simulink model "ControlSystemDesign"  (R2020a)
settings: Solver=VariableStepAuto  StartTime=0.0  StopTime=100.0  RelTol=1e-3
values from neighbouring files (symbols this model uses):
  J = m/12*(l^2*cos(beta)^2+d^2*sin(beta)^2+w^2)    [SolarPanelMotorParams.m]
  Kd = 5    [SolarPanelMotorParams.m]
  Kf = 0.07    [SolarPanelMotorParams.m]
  Kg = 2000    [SolarPanelMotorParams.m]
  Kt = 0.07    [SolarPanelMotorParams.m]
  L = 1e-5    (= 1e-05)    [SolarPanelMotorParams.m]
  R = 10    [SolarPanelMotorParams.m]
libraries: simulink x1
settings Model: Creator=aztaa  LastModifiedBy=aztaa

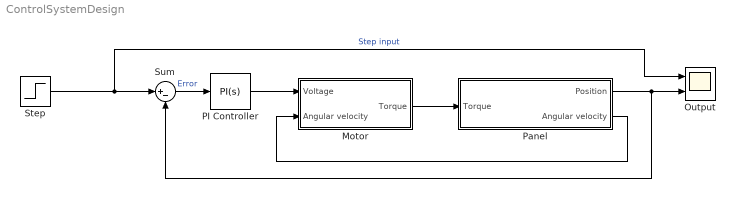
== system ControlSystemDesign ==
  Motor : Subsystem
  Output : Scope  NumInputPorts=2
  PI Controller : simulink/Continuous/PID Controller  Controller=PI  Form=Parallel  TimeDomain=Continuous-time  UseExternalTs=off  SampleTime=-1  IntegratorMethod=Forward Euler  FilterMethod=Forward Euler  ControllerParametersSource=internal  P=300  I=200  D=0  UseFilter=on  N=100  TunerSelectOption=Transfer Function Based (PID Tuner App)  InitialConditionSource=internal  InitialConditionForIntegrator=0  InitialConditionForFilter=0  DifferentiatorICPrevScaledInput=0  ExternalReset=none  TrackingMode=off  Kt=1  LimitOutput=off  UpperSaturationLimit=inf  LowerSaturationLimit=-inf  LinearizeAsGain=on  AntiWindupMode=none  Kb=1  POutMin=[]  POutMax=[]  IOutMin=[]  IOutMax=[]  DOutMin=[]  DOutMax=[]  NOutMin=[]  NOutMax=[]  SumOutMin=[]  SumOutMax=[]  SaturationOutMin=[]  SaturationOutMax=[]  PParamMin=[]  PParamMax=[]  IParamMin=[]  IParamMax=[]  DParamMin=[]  DParamMax=[]  NParamMin=[]  NParamMax=[]  KbParamMin=[]  KbParamMax=[]  KtParamMin=[]  KtParamMax=[]  KbOutMin=[]  KbOutMax=[]  KtOutMin=[]  KtOutMax=[]  IntegratorOutMin=[]  IntegratorOutMax=[]  FilterOutMin=[]  FilterOutMax=[]  SumI1OutMin=[]  SumI1OutMax=[]  SumI2OutMin=[]  SumI2OutMax=[]  SumI3OutMin=[]  SumI3OutMax=[]  SumI4OutMin=[]  SumI4OutMax=[]  SumDOutMin=[]  SumDOutMax=[]  DifferentiatorOutMin=[]  DifferentiatorOutMax=[]  FilterDiffOutCoefMin=[]  FilterDiffOutCoefMax=[]  ReciprocalOutMin=[]  ReciprocalOutMax=[]  SumDenOutMin=[]  SumDenOutMax=[]  SumNumOutMin=[]  SumNumOutMax=[]  DivideOutMin=[]  DivideOutMax=[]  UdiffTsProdOutMin=[]  UdiffTsProdOutMax=[]  NTsProdOutMin=[]  NTsProdOutMax=[]  UintegralTsProdOutMin=[]  UintegralTsProdOutMax=[]  UngainTsProdOutMin=[]  UngainTsProdOutMax=[]  IntegratorContinuousStateAttributes=''  IntegratorStateMustResolveToSignalObject=off  IntegratorRTWStateStorageClass=Auto  FilterContinuousStateAttributes=''  FilterStateMustResolveToSignalObject=off  FilterRTWStateStorageClass=Auto  ParallelPVariant=InternalParameters  IdealPVariant=Disabled  IVariant=InternalParameters  DVariant=Disabled  IntegratorVariant=Continuous  SatVariant=Disabled  AWVariant=Passthrough  PCopyVariant=Disabled  TRVariant=Disabled  FdbkBlocksVariant=Forward  IdealPFdbkVariant=Disabled  SatFdbkVariant=Disabled  DerivativeFilterVariant=Disabled  NVariant=Disabled  NCopyVariant=Disabled_SignalSpec  FilterICVariant=Disabled  IntegratorICVariant=InternalICs  ExternalResetVariant=Disabled  TRSumVariant=Passthrough  SumFdbkVariant=Disabled  SumVariant=Sum_PI  TsampFilterVariant=InternalTs  TsampNgainVariant=Passthrough  TsampIntegralVariant=Passthrough
  Panel : Subsystem
  Step : Step  SampleTime=0
  Sum : Sum  Inputs=|+-
  wires:
  Panel/1(Position) -> Output/2, Sum/2
  Motor/1(Torque) -> Panel/1(Torque)
  Panel/2(Angular velocity) -> Motor/2(Angular velocity)
  PI Controller/1 -> Motor/1(Voltage)
  Sum/1 -> PI Controller/1  "Error"
  Step/1 -> Output/1, Sum/1  "Step input"

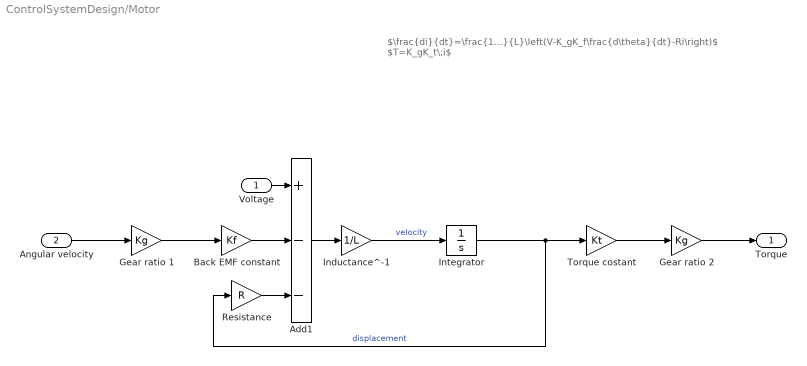
== system ControlSystemDesign/Motor ==
  note: $\frac{di}{dt}=\frac{1}{L}\left(V-K_gK_f\frac{d\theta}{dt}-Ri\right)$
      | $T=K_gK_t\;i$
  Voltage : Inport
  Angular velocity : Inport  Port=2
  Add1 : Sum  Inputs=+--
  Back EMF constant : Gain  Gain=Kf
  Gear ratio 1 : Gain  Gain=Kg
  Gear ratio 2 : Gain  Gain=Kg
  Inductance^-1 : Gain  Gain=1/L
  Integrator : Integrator
  Resistance : Gain  Gain=R
  Torque costant : Gain  Gain=Kt
  Torque : Outport
  wires:
  Add1/1 -> Inductance^-1/1
  Back EMF constant/1 -> Add1/2
  Voltage/1 -> Add1/1
  Integrator/1 -> Torque costant/1, Resistance/1  "displacement"
  Inductance^-1/1 -> Integrator/1  "velocity"
  Gear ratio 1/1 -> Back EMF constant/1
  Torque costant/1 -> Gear ratio 2/1
  Resistance/1 -> Add1/3
  Gear ratio 2/1 -> Torque/1
  Angular velocity/1 -> Gear ratio 1/1

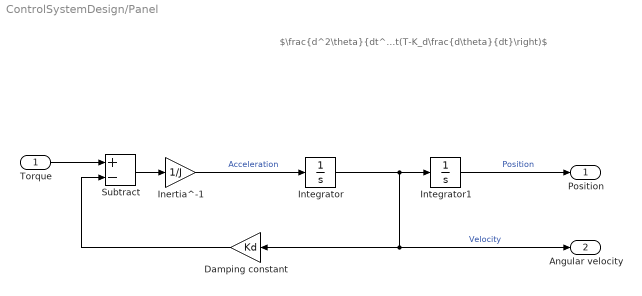
== system ControlSystemDesign/Panel ==
  note: $\frac{d^2\theta}{dt^2}=\frac{1}{J}\left(T-K_d\frac{d\theta}{dt}\right)$
  Torque : Inport
  Damping constant : Gain  Gain=Kd
  Inertia^-1 : Gain  Gain=1/J
  Integrator : Integrator
  Integrator1 : Integrator
  Subtract : Sum  Inputs=+-
  Position : Outport
  Angular velocity : Outport  Port=2
  wires:
  Damping constant/1 -> Subtract/2
  Torque/1 -> Subtract/1
  Integrator/1 -> Integrator1/1, Angular velocity/1, Damping constant/1  "Velocity"
  Subtract/1 -> Inertia^-1/1
  Inertia^-1/1 -> Integrator/1  "Acceleration"
  Integrator1/1 -> Position/1  "Position"
